simulink model "GHV_open_air_ang_trajectory_design_toolbox"  (R2023b)
settings: Solver=VariableStepAuto  StartTime=0.0  StopTime=130  FixedStep=0.0000001  MaxStep=0.001  RelTol=1e-3
InitFcn:
  | run('init.m')
undefined symbols (not defined in the file or in its folder): GHV_cfg
libraries: simulink_extras x3, aerolibasang x2, aerolibadyn x1, aerolibatmos2 x1
settings Model: SimulationMode=accelerator  Creator=Admin  LastModifiedBy=Admin
settings SolverCC: AllowMultiTaskInputOutput=on  ZeroCrossControl=EnableAll  ZeroCrossAlgorithm=Adaptive  AutoInsertRateTranBlk=on

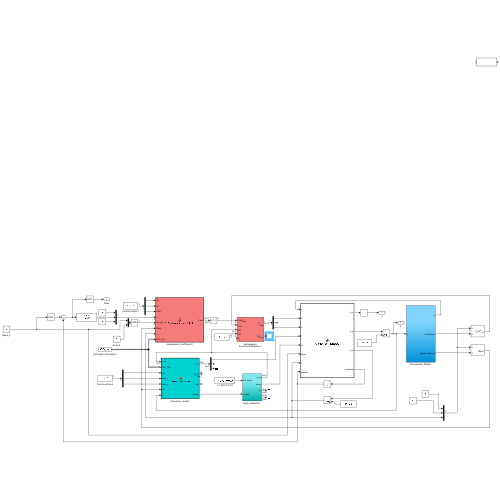
[thumbnail: Simulink's stored preview of the top-level diagram]
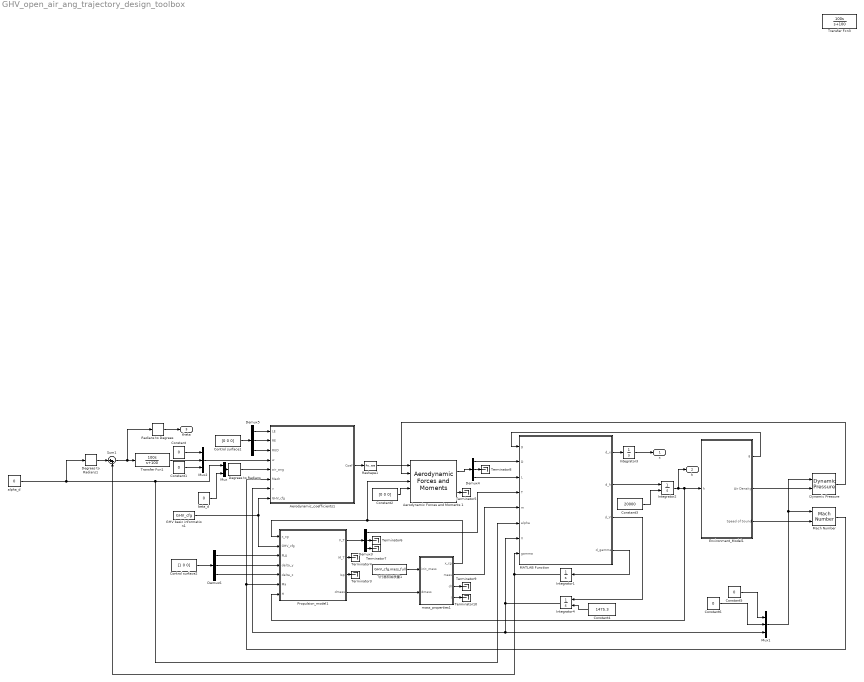
== system GHV_open_air_ang_trajectory_design_toolbox ==
  Aerodynamic Forces and Moments 1 : aerolibadyn/Aerodynamic Forces and Moments   inputAxes=Body  outputForceAxes=Wind  outputMomentAxes=Body  S=GHV_cfg.s_ref  b=GHV_cfg.b_ref  cbar=GHV_cfg.c_ref
  Aerodynamic_coefficients1 : MATLAB Function  TreatAsAtomicUnit=on
  Constant{,1,5..6} (4 alike) : Constant  Value=0
  Constant2 : Constant  Value=[0 0 0]
  Constant3 : Constant  Value=20000
  Constant4 : Constant  Value=1475.3
  Control surface1 : Constant  Value=[0 0 0]
  Control surface2 : Constant  Value=[1 0 0]
  Degrees to Radians : simulink_extras/Transformations/Degrees to Radians
  Degrees to Radians1 : simulink_extras/Transformations/Degrees to Radians
  Demux{3..6} (4 alike) : Demux  Outputs=3
  Dynamic Pressure : aerolibasang/Dynamic Pressure
  Environment_Model1 : Subsystem
  GHV basic information1 : Constant  Value=GHV_cfg  VectorParams1D=off  OutDataTypeStr=Bus: slBus1
  Integrator1 : Integrator
  Integrator2 : Integrator  InitialConditionSource=external
  Integrator3 : Integrator
  Integrator4 : Integrator  InitialConditionSource=external
  MATLAB Function : MATLAB Function  TreatAsAtomicUnit=on
  Mach Number : aerolibasang/Mach Number
  Mux : Mux  Inputs=2
  Mux1 : Mux  Inputs=3
  Mux2 : Mux  Inputs=3
  Propulsion_model1 : MATLAB Function  TreatAsAtomicUnit=on
  Radians to Degrees : simulink_extras/Transformations/Radians to Degrees
  Reshape1 : Reshape
  Sum1 : Sum  Inputs=|++
  Terminator{3..10} (8 alike) : Terminator
  Transfer Fcn1 : TransferFcn  Numerator=[100 0]  Denominator=[1 100]
  Transfer Fcn3 : TransferFcn  Numerator=[100 0]  Denominator=[1 100]
  alpha_d : Constant  Value=0  VectorParams1D=off
  beta_d : Constant  Value=0  VectorParams1D=off
  mass_properties1 : Subsystem
  飞行器初始质量1 : Constant  Value=GHV_cfg.mass_full
  x : Outport
  h : Outport  Port=2
  theta : Outport  Port=3
  wires:
  MATLAB Function/4(d_gamma) -> Integrator1/1
  MATLAB Function/2(d_h) -> Integrator2/1
  MATLAB Function/1(d_x) -> Integrator3/1
  Aerodynamic_coefficients1/1(Coef) -> Reshape1/1
  Propulsion_model1/4(dmass) -> mass_properties1/2(dmass)
  Reshape1/1 -> Aerodynamic Forces and Moments 1/1
  mass_properties1/1(x_cg) -> Propulsion_model1/1(x_cg), Aerodynamic Forces and Moments 1/3
  Constant2/1 -> Aerodynamic Forces and Moments 1/4
  Propulsion_model1/3(Isp) -> Terminator3/1
  Propulsion_model1/2(M_T) -> Terminator4/1
  Aerodynamic Forces and Moments 1/2 -> Terminator5/1
  Propulsion_model1/1(F_T) -> Demux3/1
  Demux3/2 -> Terminator6/1
  Demux3/3 -> Terminator7/1
  Demux3/1 -> MATLAB Function/4(T)
  Aerodynamic Forces and Moments 1/1 -> Demux4/1
  Demux4/2 -> Terminator8/1
  Demux4/1 -> MATLAB Function/2(D)
  Demux4/3 -> MATLAB Function/3(L)
  mass_properties1/2(mass) -> MATLAB Function/5(m)
  mass_properties1/3(dI) -> Terminator9/1
  mass_properties1/4(I) -> Terminator10/1
  飞行器初始质量1/1 -> mass_properties1/1(init_mass)
  GHV basic information1/1 -> Aerodynamic_coefficients1/8(GHV_cfg), Propulsion_model1/2(GHV_cfg)
  Demux5/3 -> Aerodynamic_coefficients1/3(RUD)
  Demux5/1 -> Aerodynamic_coefficients1/1(LE)
  Demux5/2 -> Aerodynamic_coefficients1/2(RE)
  Control surface1/1 -> Demux5/1
  Control surface2/1 -> Demux6/1
  Demux6/1 -> Propulsion_model1/3(PLA)
  Demux6/2 -> Propulsion_model1/4(delta_y)
  Demux6/3 -> Propulsion_model1/5(delta_z)
  Integrator1/1 -> Sum1/2, MATLAB Function/8(gamma)
  Integrator4/1 -> MATLAB Function/7(V), Mux1/3, Aerodynamic_coefficients1/7(v)
  Integrator2/1 -> h/1, Environment_Model1/1(h), Propulsion_model1/7(H)
  Environment_Model1/1(g) -> MATLAB Function/1(g)
  Integrator3/1 -> x/1
  MATLAB Function/3(d_V) -> Integrator4/1
  Environment_Model1/2(Air Density) -> Dynamic Pressure/2
  Environment_Model1/3(Speed of Sound) -> Mach Number/2
  Mach Number/1 -> Propulsion_model1/6(Ma), Aerodynamic_coefficients1/6(Mach)
  Dynamic Pressure/1 -> Aerodynamic Forces and Moments 1/2
  Constant3/1 -> Integrator2/2
  Degrees to Radians/1 -> Aerodynamic_coefficients1/5(air_ang)
  alpha_d/1 -> Degrees to Radians1/1, Mux/1, MATLAB Function/6(alpha)
  Mux/1 -> Degrees to Radians/1
  beta_d/1 -> Mux/2
  Transfer Fcn1/1 -> Mux2/2
  Mux2/1 -> Aerodynamic_coefficients1/4(w)
  Constant1/1 -> Mux2/3
  Constant/1 -> Mux2/1
  Constant4/1 -> Integrator4/2
  Sum1/1 -> Transfer Fcn1/1, Radians to Degrees/1
  Mux1/1 -> Mach Number/1, Dynamic Pressure/1
  Constant5/1 -> Mux1/1
  Constant6/1 -> Mux1/2
  Degrees to Radians1/1 -> Sum1/1
  Radians to Degrees/1 -> theta/1

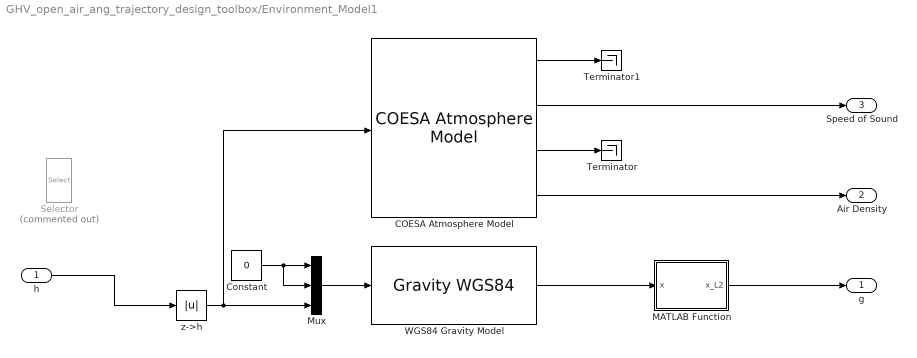
== system GHV_open_air_ang_trajectory_design_toolbox/Environment_Model1 ==
  h : Inport
  COESA Atmosphere Model : aerolibatmos2/COESA Atmosphere Model  units=Metric (MKS)  spec=1976 COESA-extended U.S. Standard Atmosphere  model=Profile  profile_var=High temperature  profile_percent=1%  profile_alt=5 km (16404 ft)  envelope_var=High temperature  envelope_percent=1%  action=Warning
  Constant : Constant  Value=0
  MATLAB Function : MATLAB Function  TreatAsAtomicUnit=on
  Mux : Mux  Inputs=3
  Selector : Selector  Commented=on  InputPortWidth=3  IndexOptions=Index vector (dialog)  Indices=[3]  OutputSizes=1
  Terminator : Terminator
  Terminator1 : Terminator
  "WGS84 Gravity Model  " : GravityWGS84  action=Error
  z->h : Abs  SaturateOnIntegerOverflow=off
  g : Outport
  Air Density : Outport  Port=2
  Speed of Sound : Outport  Port=3
  wires:
  "WGS84 Gravity Model  "/1 -> MATLAB Function/1(x)
  Constant/1 -> Mux/2, Mux/1
  z->h/1 -> COESA Atmosphere Model/1, Mux/3
  Mux/1 -> "WGS84 Gravity Model  "/1
  COESA Atmosphere Model/1 -> Terminator1/1
  COESA Atmosphere Model/2 -> Speed of Sound/1
  COESA Atmosphere Model/3 -> Terminator/1
  COESA Atmosphere Model/4 -> Air Density/1
  MATLAB Function/1(x_L2) -> g/1
  h/1 -> z->h/1

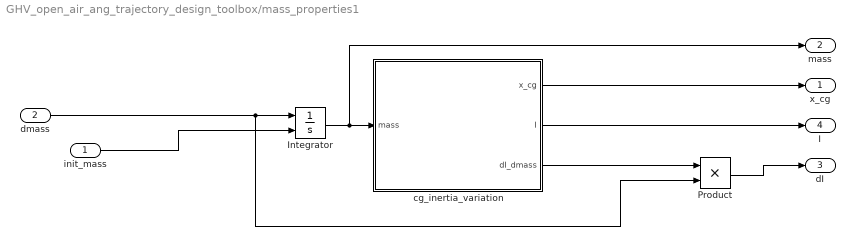
== system GHV_open_air_ang_trajectory_design_toolbox/mass_properties1 ==
  init_mass : Inport
  dmass : Inport  Port=2
  Integrator : Integrator  InitialConditionSource=external
  Product : Product
  cg_inertia_variation : MATLAB Function  TreatAsAtomicUnit=on
  x_cg : Outport
  mass : Outport  Port=2
  dI : Outport  Port=3
  I : Outport  Port=4
  wires:
  Integrator/1 -> mass/1, cg_inertia_variation/1(mass)
  init_mass/1 -> Integrator/2
  cg_inertia_variation/3(dI_dmass) -> Product/1
  dmass/1 -> Product/2, Integrator/1
  cg_inertia_variation/2(I) -> I/1
  cg_inertia_variation/1(x_cg) -> x_cg/1
  Product/1 -> dI/1

== matlab function GHV_open_air_ang_trajectory_design_toolbox/MATLAB Function ==
  data: g input; D input; L input; d_x output; d_h output; d_V output; d_gamma output; T input; m input; alpha input; V input; gamma input
function [d_x, d_h, d_V, d_gamma] = S_three_dof_trajectory(g, D, L, T, m, alpha, V, gamma)

    [d_V, d_gamma, d_x, d_h] = three_dof_trajectory(T, D, L, alpha, m, g, V, gamma);


end

== matlab function GHV_open_air_ang_trajectory_design_toolbox/Aerodynamic_coefficients1 ==
  data: LE input; Coef output; RE input; RUD input; w input; air_ang input; Mach input; v input; GHV_cfg input
function Coef = S_Aerodynamic_coefficients(LE, RE, RUD, w, air_ang, Mach, v, GHV_cfg)
    Coef = zeros(6, 1);
    Coef = Aerodynamic_coefficients(LE, RE, RUD, air_ang, v, w, Mach, GHV_cfg);

end

== matlab function GHV_open_air_ang_trajectory_design_toolbox/Propulsion_model1 ==
  data: x_cg input; GHV_cfg input; PLA input; delta_y input; delta_z input; Ma input; H input; F_T output; M_T output; Isp output; dmass output
function  [F_T, M_T, Isp, dmass] = S_Propulsion_model(x_cg, GHV_cfg, PLA, delta_y, delta_z, Ma, H)
    F_T = zeros(3, 1); %#ok<PREALL>
    M_T = zeros(3, 1); %#ok<PREALL>
   [F_T, M_T, Isp, dmass] = Propulsion_model(PLA, H, Ma, delta_y, delta_z, GHV_cfg, x_cg);

end

== matlab function GHV_open_air_ang_trajectory_design_toolbox/mass_properties1/cg_inertia_variation ==
  data: mass input; x_cg output; I output; dI_dmass output
function [x_cg, I, dI_dmass] = S_cg_inertia_variation(mass)

     [x_cg, I, dI_dmass] = cg_inertia_variation(mass);
     
end

== matlab function GHV_open_air_ang_trajectory_design_toolbox/Environment_Model1/MATLAB Function ==
  data: x input; x_L2 output
function x_L2 = S_L2Norm(x)

    x_L2 = L2Norm(x);

end
